simulink model "ALGO_TrajTrack_MPC_new"  (R2023a)
settings: Solver=VariableStepAuto  StartTime=0.0  StopTime=60  RelTol=1e-3
StopFcn:
  | CompareSimResult_anti_rollover
libraries: simulink x7, slpidlib x1, Solver_SF x1
(part 2 of 2)

== matlab function ALGO_TrajTrack_MPC_new/DiffBrkCtrller ==
  data: vx input; refState output; delta input; stateMPC input; errState output; extM output
function [refState,errState,extM]=RefModel_5DOF(vx, delta, stateMPC)
    %% 获取真实的状态
    realState=TruckSimInput(stateMPC);
    %% 初始状态定义
    %要记得设置本模块的采样时间哦
    persistent Ts                             %采样时间
    persistent  vy10 df10 F10 dF10 Y10 X10 f10 %牵引车状态变量
    persistent  vy20 df20 F20 dF20 Y20 X20 f20 %半挂车状态变量
    if isempty(vy10)
       Ts=0.01;%采样时间
       %初始化状态量
       vy10=0; df10=0;F10=0;dF10=0; Y10=0;X10=0;f10=0;
       vy20=0; df20=0;F20=0;dF20=0; Y20=0;X20=-5.638315;f20=0;
    end
    %% 定义动力学模型参数
    persistent a b c d e                    %轴距纵向几何参数
    persistent h1 h2 hc1 hc2                %质心至侧倾轴线距离
                                            %铰接点至侧倾轴线距离
    persistent m1 m2 m1s m2s g;g=9.806;
    persistent I1zz I1xx I1xz I2zz I2xx I2xz %惯性参量
    persistent k1 k2 k3                      %线性轮胎模型参数
    persistent kr1 kr2 c1 c2 k12             %悬架模型参数
    if isempty(a)
        %车辆模型参数
        L1=(5+6.27)/2;L2=(10.15+11.5)/2;       %轴距平均
        a=1.385;b=L1-a;c=5.635-a;e=5.5;d=L2-e; %纵向几何
        hm1s=1.02; %牵引车质心高度
        hm2s=1.58; %50%充液率时半挂车质心高度
        hhitch=1.1;%交接点高度
        hroll1=0.2314;hroll2=0.9630;                     %侧倾中心高度
        h1=hm1s-hroll1;h2=hm2s-hroll2;hc1=hhitch-hroll1;hc2=hhitch-hroll2;%高度几何
        m1s=6310;m1=m1s+570+785*2;             %牵引车质量
        % m2s=5925;m2=m2s+665*2;                 %半挂车空载质量
        m2s=20387;m2=m2s+665*2;
        I1xx=6879;I1xz=130;I1zz=19665;         %牵引车惯量
        % I2xx=9960;I2xz=0;I2zz=179992;          %半挂车惯量
        I2xx=34652;I2xz=0;I2zz=331380;
        %轮胎模型参数
        k1=-37e4;k2=-82e4;k3=-80e4;             %侧偏刚度
        kr1=18.7e5;kr2=9.14e5;k12=68.3e5;             %侧倾刚度
        c1=64.4e3;c2=197.7e3;                        %悬架等效阻尼
    end
    %% 定义线性动力学模型
    vy1=vy10;df1=df10;F1=F10;dF1=dF10;Y1=Y10;X1=X10;f1=f10;
    vy2=vy20;df2=df20;F2=F20;dF2=dF20;Y2=Y20;X2=X20;f2=f20;
    vx1=vx(1);vx2=vx(2);
    %线性车辆动力学模型
    % M*dX = A0*X + B0*u
    m14=-m1s*h1*c-I1xz;
    m21=m1*vx1*hc1-m1s*h1*vx1;
    m24=I1xx+2*m1s*h1^2-m1s*h1*hc1;
    m55=m2*vx2*hc2-m2s*h2*vx2;
    m58=I2xx+2*m2s*h2^2-m2s*h2*hc2;
    
    M=[m1*vx1*c, I1zz, 0,   m14,     0,        0,   0,     0;
        m21,    -I1xz, 0,   m24,     0,        0,   0,     0;
       m1*vx1,      0, 0, -m1s*h1, m2*vx2,     0,   0, -m2s*h2;
         0,         0, 0,     0,  m2*vx2*e, -I2zz,  0, I2xz-m2s*h2*e;
         0,         0, 0,     0,    m55,    -I2xz,  0,    m58;
         1,    -c/vx1, 0, -hc1/vx1,  -1,   -e/vx2,  0, hc2/vx2;
         0,         0, 1,     0,     0,        0,   0,     0;
         0,         0, 0,     0,     0,        0,   1,     0   ];
     
    a11 = (c+a)*k1 + (c-b)*k2;
    a12 = a*(c+a)*k1/vx1 - b*(c-b)*k2/vx1 - m1*vx1*c;
    a22 = (a*k1-b*k2)*hc1/vx1 + (m1s*h1-m1*hc1)*vx1;
    a23 = m1s*g*h1 - kr1 -k12;
    a32 = (a*k1-b*k2)/vx1 - m1*vx1;
    a36 = -d*k3/vx2 - m2*vx2;
    a46 = -d*(e+d)*k3/vx2 - m2*vx2*e;
    a56 = (m2s*h2-m2*hc2)*vx2 - d*k3*hc2/vx2;
    a57 = m2s*g*h2 - kr2 -k12;
    %  X=   b1     df1    F1  dF1        b2  df2, F2   dF2 
    Acm0=[ a11,    a12,    0,   0,       0,   0,  0,    0;
        (k1+k2)*hc1, a22,  a23, -c1,       0,   0, k12,   0;
         k1+k2,     a32,    0,   0,      k3,  a36, 0,    0;
            0,       0,     0,   0, (e+d)*k3, a46, 0,    0;
            0,       0,    k12,  0,   k3*hc2, a56, a57, -c2;
            0,      -1,     0,   0,       0,   1,  0,    0;
            0,       0,     0,   1,       0,   0,  0,    0;
            0,       0,     0,   0,       0,   0,  0,    1   ];
        
    Bcm0 = [-(c+a)*k1, -k1*hc1, -k1, 0, 0, 0, 0, 0]';
    
    Acm = M \ Acm0;
    Bcm = M \ Bcm0;
    Ecm = M \ [1 0 0 0 0 0 0 0; 0 0 0 -1 0 0 0 0]';
    refState = -inv(Acm)*Bcm*delta;
    errState = realState(1:8) - refState;
    %% 进行LQR差动制动计算
    Q =1000*diag([1,10,20,100,1,10,50,200]);
    R = 0.001*diag([5,5]);
    K0 = zeros(2,8);
    K = zeros(2,8);
    coder.extrinsic("lqr")
    K0(1:2,1:8) = lqr(Acm,Ecm,Q,R);
    K(1:2,1:8) = K0;
    extM = -K*reshape(errState,8,1);
    
    
    
     %% 增广状态量 并转变bi为vyi
     
     Trans=diag([vx1,1,1,1,vx2,1,1,1]);
     Ac=[Trans*Acm/Trans,zeros(8,8);            %增广状态量后的矩阵
         0,1,0,0,0,0,0,0,0,0,0,0,0,0,0,0;
         0,0,0,0,0,1,0,0,0,0,0,0,0,0,0,0;
         zeros(2,16);
         cos(f1),0,0,0,0,0,0,0,0,0,sin(f1),0,0,0,0,0;
        -sin(f1),0,0,0,0,0,0,0,0,0,cos(f1),0,0,0,0,0;
         0,0,0,0,cos(f2),0,0,0,0,0,0,sin(f2),0,0,0,0;
        0,0,0,0,-sin(f2),0,0,0,0,0,0,cos(f2),0,0,0,0  ];
    
     Bc=[Trans*Bcm;zeros(8,1)] ;
     
     %% 离散化线性模型
     [A,B]=c2d_zoh(Ac,Bc,Ts);             %离散化线性模型
     
    %       1   2    3    4   5    6    7    8    9  10   11  12  13  14 15 16
    % dX=[dvy1;ddf1;dF1;ddF1;dvy2;ddf2;dF2;ddF2;df1;df2;dvx1;dvx2;dY1;dX2;dY2;dX2];
    %维度：14×1 
    
    %% 更新状态量
    %组装状态量
    state0=[vy1,df1,F1,dF1,vy2,df2,F2,dF2,f1,f2,vx1,vx2,Y1,X1,Y2,X2]';
    state=A*state0+B*delta;  %进行下一步更新
    
    %% 拆解状态量并为下一步计算保存
    
    X10=state(14);Y10=state(13);vy10=state(1);df10=state(2);
    F10=state(3);dF10=state(4);f10=state(9);
    X20=state(16);Y20=state(15);vy20=state(5);df20=state(6);
    F20=state(7);dF20=state(8);f20=state(10);
    


end


%% 子函数：输入单位转换*******************************
% 状态量：state==[vy1,df1,F1,dF1,vy2,df2,F2,dF2,...
%                 th,dth,f1,f2,vx1,vx2,Y1,X1,Y2,X2]';18×1 Nx=18
function state=TruckSimInput(u)
    vy1=u(1)/3.6;
    df1=u(2)/180*pi;
    F1=u(3)/180*pi;
    dF1=u(4)/180*pi;
    vy2=u(5)/3.6;
    df2=u(6)/180*pi;
    F2=u(7)/180*pi;
    dF2=u(8)/180*pi;
    th=u(9);
    dth=u(10);
    f1=u(11)/180*pi;
    f2=u(12)/180*pi;
    vx1=u(13)/3.6;
    vx2=u(14)/3.6;
    Y1=u(15);
    X1=u(16);
    Y2=u(17);
    X2=u(18);
    state=[vy1,df1,F1,dF1,vy2,df2,F2,dF2,...
          th,dth,f1,f2,vx1,vx2,Y1,X1,Y2,X2]';%18×1 Nx=18
end

== matlab function ALGO_TrajTrack_MPC_new/DiffBrk ==
  data: extM input; PresBrk output; refState input; stateMPC input
function PresBrk = DiffBrk(extM,refState,stateMPC)
    PresBrk = zeros(10,1); % 初始化制动压力指令
    realState = TruckSimInput(stateMPC);
    dyaw1 = realState(2); % 提取实际状态量
    dyaw2 = realState(6); 
    dyaw1r = refState(2); % 提取参考状态量
    dyaw2r = refState(6);
    
    thred = 1e-2;
    % 牵引车的制动
    if dyaw1 > thred
        if dyaw1r > thred
            if dyaw1r > (dyaw1+thred)
                idx1 = 3;
            elseif dyaw1r < (dyaw1-thred)
                idx1 = 2;
            else
                idx1 = 0;
            end
        elseif dyaw1r < -thred
            idx1 = 2;
        else
            idx1 = 2;
        end
    elseif dyaw1 < -thred
        if dyaw1r > thred
            idx1 = 1;
        elseif dyaw1r < -thred
            if dyaw1r > (dyaw1+thred)
                idx1 = 1;
            elseif dyaw1r < (dyaw1-thred)
                idx1 = 4;
            else
                idx1 = 0;
            end
        else
            idx1 = 1;
        end
    else
        if dyaw1r > thred
            idx1 = 3;
        elseif dyaw1r < -thred
            idx1 = 4;
        else
            idx1 = 0;
        end
    end
    
    % 半挂车的制动
    if dyaw2 > thred
        if dyaw2r > thred
            if dyaw2r > (dyaw2+thred)
                idx2 = 5;
            elseif dyaw2r < (dyaw2-thred)
                idx2 = 6;
            else
                idx2 = 0;
            end
        elseif dyaw2r < -thred
            idx2 = 6;
        else
            idx2 = 6;
        end
    elseif dyaw2 < -thred
        if dyaw2r > thred
            idx2 = 5;
        elseif dyaw2r < -thred
            if dyaw2r > (dyaw2+thred)
                idx2 = 5;
            elseif dyaw2r < (dyaw2-thred)
                idx2 = 6;
            else
                idx2 = 0;
            end
        else
            idx2 = 5;
        end
    else
        if dyaw2r > thred
            idx2 = 5;
        elseif dyaw2r < -thred
            idx2 = 6;
        else
            idx2 = 0;
        end
    end
    
    switch idx1
        case 1
            PresBrk(1) = abs(extM(1));
        case 2
            PresBrk(6) = abs(extM(1));
        case 3
            PresBrk([2 3]) = abs(extM(1));
        case 4
            PresBrk([7 8]) = abs(extM(1));
    end
    switch idx2
        case 5
            PresBrk([4 5]) = abs(extM(2));
        case 6
            PresBrk([9 10]) = abs(extM(2));
    end
end


%% 子函数：输入单位转换*******************************
% 状态量：state==[vy1,df1,F1,dF1,vy2,df2,F2,dF2,...
%                 th,dth,f1,f2,vx1,vx2,Y1,X1,Y2,X2]';18×1 Nx=18
function state=TruckSimInput(u)
    vy1=u(1)/3.6;
    df1=u(2)/180*pi;
    F1=u(3)/180*pi;
    dF1=u(4)/180*pi;
    vy2=u(5)/3.6;
    df2=u(6)/180*pi;
    F2=u(7)/180*pi;
    dF2=u(8)/180*pi;
    th=u(9);
    dth=u(10);
    f1=u(11)/180*pi;
    f2=u(12)/180*pi;
    vx1=u(13)/3.6;
    vx2=u(14)/3.6;
    Y1=u(15);
    X1=u(16);
    Y2=u(17);
    X2=u(18);
    state=[vy1,df1,F1,dF1,vy2,df2,F2,dF2,...
          th,dth,f1,f2,vx1,vx2,Y1,X1,Y2,X2]';%18×1 Nx=18
end
